simulink model "GaussNoise"  (Simulink 8.2)
settings: Solver=ode45  StartTime=0.0  StopTime=10  RelTol=1e-3
undefined symbols (not defined in the file or in its folder): fdesignblkfcn, gcbh, magnitude
libraries: dspxfrm3 x1, commnoisgen2 x1
settings Model: Creator=Yi_Liu  LastModifiedBy=Yi_Liu
settings DataIOCC: SignalLoggingSaveFormat=Dataset
settings OptimizationCC: ExpressionDepthLimit=128
settings DebuggingCC: FcnCallInpInsideContextMsg=EnableAllAsError  StateNameClashWarn=none
settings GRTTargetCC: CombineOutputUpdateFcns=on  GRTInterface=off

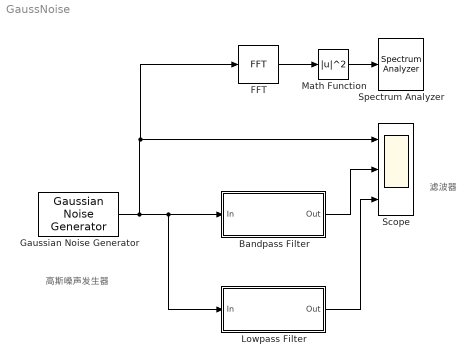
== system GaussNoise ==
  note: 滤波器
  note: 高斯噪声发生器
  Bandpass Filter : Subsystem  DialogController=fdesignblkfcn  DialogControllerArgs=DataTag1  InitFcn=fdesignblkfcn(gcbh, {'InitFcn'});  mask(Bandpass Filter){}
      mask help: Design a bandpass filter
      settings: CopyFcn=fdesignblkfcn(gcbh, {'CopyFcn'});
      mask Help: helpview(mapfilelocation('dsp'), 'dspbandpassfilter');
      mask Display: disp('Bandpass');
  FFT : dspxfrm3/FFT  CompMethod=Table lookup  TableOpt=NEW  TableOptActive=Speed  BitRevOrder=off  InheritFFTLength=on  FFTLength=64  RowConvenienceOn=on  FFTImplementation=Auto  SkipNorm=off  firstCoeffDataTypeStr=Inherit: Same word length as input  firstCoeffLastDataTypeStr=Inherit: Same word length as input  outputMin=[]  outputMax=[]  roundingMode=Floor  overflowMode=off
  Gaussian Noise Generator : commnoisgen2/Gaussian Noise Generator  m=0  d=1  s=61  Ts=0.01  frameBased=off  sampPerFrame=1  orient=off  outDataType=double
  Lowpass Filter : Subsystem  DialogController=fdesignblkfcn  DialogControllerArgs=DataTag3  InitFcn=fdesignblkfcn(gcbh, {'InitFcn'});  mask(Lowpass Filter){}
      mask help: Design a lowpass filter
      settings: CopyFcn=fdesignblkfcn(gcbh, {'CopyFcn'});
      mask Help: helpview(mapfilelocation('dsp'), 'dsplowpassfilter');
      mask Display: disp('Lowpass')
  Math Function : Math  Operator=magnitude^2  SaturateOnIntegerOverflow=on
  Scope : Scope  NumInputPorts=3
      settings: YMin=-5~-5~-5  YMax=5~5~5
  Spectrum Analyzer : SpectrumAnalyzer  ScopeSpecification=DataTag4
      settings: CopyFcn=scopeextensions.ScopeBlock.onCoreBlockCopy(gcbh);  DeleteFcn=scopeextensions.ScopeBlock.callback(gcbh, 'onBlockDelete');  PreSaveFcn=scopeextensions.ScopeBlock.callback(gcbh, 'onModelSave');  NameChangeFcn=scopeextensions.ScopeBlock.callback(gcbh, 'onBlockRename');  DestroyFcn=scopeextensions.ScopeBlock.onBlockDestroy(gcbh)  CloseFcn=scopeextensions.ScopeBlock.callback(gcbh, 'onBlockClose');  PreDeleteFcn=scopeextensions.ScopeBlock.callback(gcbh, 'onBlockPreDelete');
  wires:
  Lowpass Filter/1(Out) -> Scope/3
  Math Function/1 -> Spectrum Analyzer/1
  Gaussian Noise Generator/1 -> FFT/1, Scope/1, Lowpass Filter/1(In), Bandpass Filter/1(In)
  Bandpass Filter/1(Out) -> Scope/2
  FFT/1 -> Math Function/1

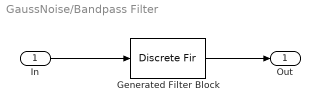
== system GaussNoise/Bandpass Filter ==
  In : Inport
  Generated Filter Block : DiscreteFir  Tag=BlockMethodSubSystem  Coefficients=[-0.00098737383861868312 -0.0010471369932502496 -0.0007031828378888037 0.00045801485136914263 0.0020881956960419959 0.0033520710058732414 0.0033548293086479376 0.0017447709431659207 -0.0009117787546616535 -0.0033248271467388752 -0.0042316157992214852 -0.0032699588763890159 -0.0013328782489038472 -3.5654340876834959e-05 -0.00052322123219949426 -0.002405798566433145 -0.0036850574987437345 -0.001982746852595503 0.0035810343080751534 0.011115970016207158 0.016429858368614787 0.01531161096956315 0.0064025240191905482 -0.0072443032881235646 -0.019269190075439483 -0.023492224608003216 -0.01780055710688656 -0.0058406244478668191 0.0049511823395518 0.0081337507714095078 0.002921310075701095 -0.0045814975456083852 -0.004993301579459891 0.0076206164286773291 0.030101417232693391 0.049800336068848067 0.050755468078788626 0.023602355426767509 -0.026545997842727889 -0.079633515365725105 -0.10914192723174915 -0.09577282041330254 -0.039007205387827537 0.040297490127018859 0.10854746800702267 0.1353523280974509 0.10854746800702267 0.040297490127018859 -0.039007205387827537 -0.09577282041330254 -0.10914192723174915 -0.079633515365725105 -0.026545997842727889 0.023602355426767509 0.050755468078788626 0.049800336068848067 0.030101417232693391 0.0076206164286773291 -0.004993301579459891 -0.0045814975456083852 0.002921310075701095 0.0081337507714095078 0.0049511823395518 -0.0058406244478668191 -0.01780055710688656 -0.023492224608003216 -0.019269190075439483 -0.0072443032881235646 0.0064025240191905482 0.01531161096956315 0.016429858368614787 0.011115970016207158 0.0035810343080751534 -0.001982746852595503 -0.0036850574987437345 -0.002405798566433145 -0.00052322123219949426 -3.5654340876834959e-05 -0.0013328782489038472 -0.0032699588763890159 -0.0042316157992214852 -0.0033248271467388752 -0.0009117787546616535 0.0017447709431659207 0.0033548293086479376 0.0033520710058732414 0.0020881956960419959 0.00045801485136914263 -0.0007031828378888037 -0.0010471369932502496 -0.00098737383861868312]  InputProcessing=Columns as channels (frame based)
  Out : Outport
  wires:
  In/1 -> Generated Filter Block/1
  Generated Filter Block/1 -> Out/1

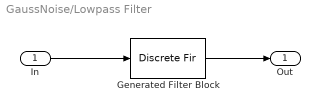
== system GaussNoise/Lowpass Filter ==
  In : Inport
  Generated Filter Block : DiscreteFir  Tag=BlockMethodSubSystem  Coefficients=[0.00082134311329856333 0.00086044183774140292 0.0011650777729448035 0.0013989605197153622 0.0014807379825975725 0.0013305171923252259 0.0008813799288182549 9.396666594465794e-05 -0.0010242764933667697 -0.0024150838129607158 -0.0039600576183871769 -0.0054879111338127784 -0.0067895716510365106 -0.0076430176358472015 -0.0078436359305586543 -0.0072403435516525732 -0.0057673738553609992 -0.0034717942727364982 -0.00052673802500832864 0.0027718950549306485 0.0060277239934803549 0.0087838441136310098 0.010579384955155792 0.011014410167142486 0.0098173087600081123 0.0069036874143378977 0.0024180557419036059 -0.0032497931384979032 -0.0094784288355618355 -0.015461211888206216 -0.020281532807071449 -0.023010985299838312 -0.02281944066888339 -0.019084347965161907 -0.011485203310779287 -7.0458864603285473e-05 0.014714050491344104 0.032040450344852957 0.050759005066959642 0.069498089116120487 0.086794001009398575 0.10123636540766748 0.11161274108764473 0.1170353898828442 0.1170353898828442 0.11161274108764473 0.10123636540766748 0.086794001009398575 0.069498089116120487 0.050759005066959642 0.032040450344852957 0.014714050491344104 -7.0458864603285473e-05 -0.011485203310779287 -0.019084347965161907 -0.02281944066888339 -0.023010985299838312 -0.020281532807071449 -0.015461211888206216 -0.0094784288355618355 -0.0032497931384979032 0.0024180557419036059 0.0069036874143378977 0.0098173087600081123 0.011014410167142486 0.010579384955155792 0.0087838441136310098 0.0060277239934803549 0.0027718950549306485 -0.00052673802500832864 -0.0034717942727364982 -0.0057673738553609992 -0.0072403435516525732 -0.0078436359305586543 -0.0076430176358472015 -0.0067895716510365106 -0.0054879111338127784 -0.0039600576183871769 -0.0024150838129607158 -0.0010242764933667697 9.396666594465794e-05 0.0008813799288182549 0.0013305171923252259 0.0014807379825975725 0.0013989605197153622 0.0011650777729448035 0.00086044183774140292 0.00082134311329856333]  InputProcessing=Columns as channels (frame based)
  Out : Outport
  wires:
  In/1 -> Generated Filter Block/1
  Generated Filter Block/1 -> Out/1
